simulink model "Seperately_excited_DC_motor"  (R2021a)
settings: Solver=VariableStepAuto  StartTime=0.0  StopTime=1  RelTol=1e-3
libraries: spsDCVoltageSourceLib x2, spsDCMachineLib x1, spspowerguiLib x1
settings Model: Creator=User  LastModifiedBy=User

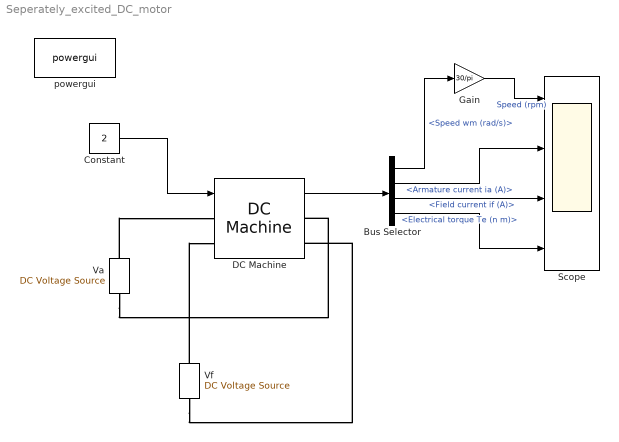
== system Seperately_excited_DC_motor ==
  Bus Selector : BusSelector  OutputSignals=Speed wm (rad/s),Armature current ia (A),Field current if (A),Electrical torque Te (n m)
  Constant : Constant  Value=2
  DC Machine : spsDCMachineLib/DC Machine  PresetModel=No  MechanicalLoad=Torque TL  FieldType=Wound  ShowDetailedParameters=on  MeasurementBus=off  RLa="[ 0.6  0.012]"  RLf="[ 240  120]"  Laf=1.8  MachineConstant=Torque constant (N.m/A)  Ke=1.8  Kt=1.8  J=1  Bm=0  Tf=0  w0=1  Ifinit=0.833333333333333  TsPowergui=0  TsBlock=-1
  Gain : Gain  Gain=30/pi
  Scope : Scope  NumInputPorts=4
  Va : spsDCVoltageSourceLib/DC Voltage Source  Amplitude=240  Measurements=None
  Vf : spsDCVoltageSourceLib/DC Voltage Source  Amplitude=200  Measurements=None
  powergui : spspowerguiLib/powergui  Priority=1  SimulationMode=Continuous  SampleTime=50e-6  frequency=60  Iterations=50  frequencyindice=0  Pbase=100e6  ErrMax=1e-4  UnitsV=kV  UnitsW=MW  buscounter=0  FunctionMessages=off  echomessages=off  EnableUseOfTLC=off  CurrentSourceSwitches=off  DisableSnubberDevices=off  DisableRonSwitches=off  DisableVfSwitches=off  DisplayEquations=off  AutomaticDiscreteSolvers=off  SolverType=Tustin/Backward Euler (TBE)  Interpol=off  ExternalGateDelay=off  methode=off  Ts=100  x0status=blocks  SPID=on  SwTol=0  HookPort=off  NonlinearTolerance=1e-4  nMaxIteration=100  ContinueOnMaxIteration=off  RestoreLinks=warning  ResistiveCurrentMeasurement=off  Frange=[0:2:500]  Ylog=off  Xlog=on  ShowGrid=off  save=off  variable=ZData  structure=0  ZoomFFT=off  StartTime=0.0  cycles=1  DisplayStyle=1  fundamental=60  FreqAxis=off  MaxFrequency=1000  frequencyindicesteady=1  RmsSteady=1  display=off
  wires:
  Constant/1 -> DC Machine/1
  DC Machine/1 -> Bus Selector/1
  Bus Selector/1 -> Gain/1  "<Speed wm (rad/s)>"
  Gain/1 -> Scope/1  "Speed (rpm)"
  Bus Selector/2 -> Scope/2  "<Armature current ia (A)>"
  Bus Selector/3 -> Scope/3  "<Field current if (A)>"
  Bus Selector/4 -> Scope/4  "<Electrical torque Te (n m)>"
  connections:
  Va/RConn1 -- DC Machine/LConn1
  Va/LConn1 -- DC Machine/RConn1
  Vf/RConn1 -- DC Machine/LConn2
  Vf/LConn1 -- DC Machine/RConn2
